simulink model "simulate_OFDM_basebandModulator"  (R2017a)
settings: Solver=VariableStepAuto  StartTime=0.0  StopTime=1  RelTol=1e-3
InitFcn:
  | Ts = 1/1000; % symbol time in serial data stream
  | N = 4; % number of orthogonal carriers
  | T = N*Ts; % symbol time in parallel data stream
libraries: commfilt2 x4, dspsrcs4 x4, commdigbbndpm3 x1, commrandsrc3 x1, dspindex x1
settings Model: Creator=prust  LastModifiedBy=prust

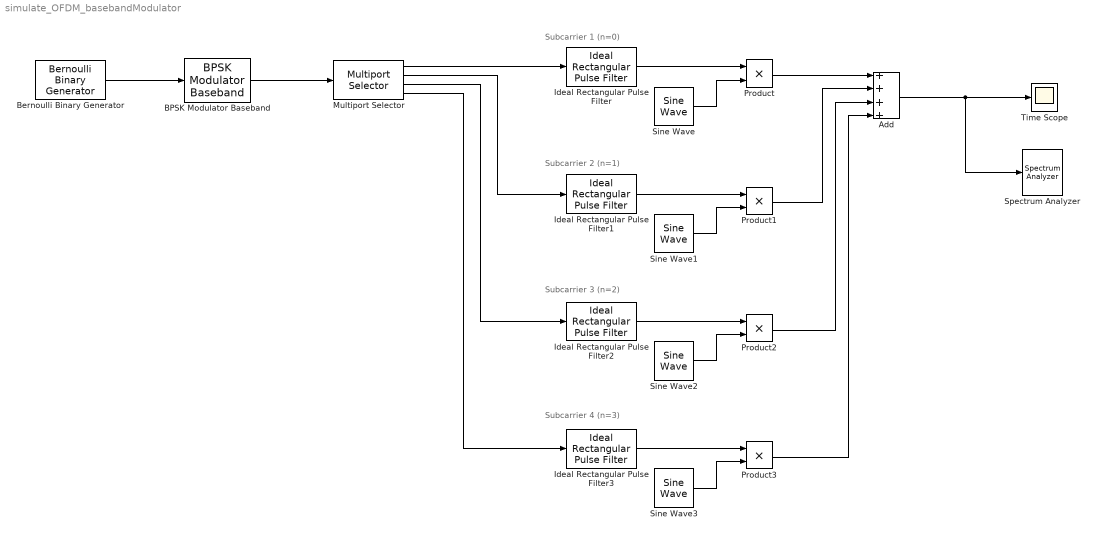
== system simulate_OFDM_basebandModulator ==
  note: Subcarrier 4 (n=3)
  note: Subcarrier 3 (n=2)
  note: Subcarrier 2 (n=1)
  note: Subcarrier 1 (n=0)
  Add : Sum  Inputs=4
  BPSK Modulator Baseband : commdigbbndpm3/BPSK Modulator Baseband  Ph=0  outDtype=double  outWordLen=16  outUDDataType=sfix(16)  outFracLenMode=Best precision  outFracLen=15  outDataTypeStr=double  outLastDataTypeStr=double
  Bernoulli Binary Generator : commrandsrc3/Bernoulli Binary Generator  ProbabilityOfZero=0.5  SeedSource=Auto  Seed=0  SampleTime=Ts  SamplesPerFrame=4  OutputDataType=double  SimulateUsing=Interpreted execution
  Ideal Rectangular Pulse Filter{,1..3} (4 alike) : commfilt2/Ideal Rectangular Pulse Filter  pulseLen=8  pulseDelay=0  InputProcessing=Columns as channels (frame based)  RateOptions=Enforce single-rate processing  sampMode=Mute  normCheck=off  normMode=Sum of samples  filterGain=1  saveAsFlag=0  roundingMode=Floor  overflowMode=off  firstCoeffDataTypeStr=Inherit: Same word length as input  firstCoeffMin=[]  firstCoeffMax=[]  firstCoeffLastDataTypeStr=Inherit: Same word length as input  outputDataTypeStr=Inherit: Same as accumulator  outputMin=[]  outputMax=[]  outputLastDataTypeStr=Inherit: Same as accumulator
      settings: SourceProductName=Communications System Toolbox  SourceProductBaseCode=CM
  Multiport Selector : dspindex/Multiport Selector  rowsOrCols=Rows  idxCellArray={ 1, 2, 3, 4 }  idxErrMode=Clip Index
  Product : Product
  "Product1 " : Product
  Product2 : Product
  Product3 : Product
  Sine Wave : dspsrcs4/Sine Wave  Amplitude=1  Frequency=-375  Phase=0  SampleMode=Discrete  OutComplex=Complex  CompMethod=Trigonometric fcn  TableSize=Speed  SampleTime=T/8  SamplesPerFrame=8  ResetState=Restart at time zero  OutputFrames=off  dataType=double  wordLen=16  udDataType=sfix(16)  fracBitsMode=Best precision  numFracBits=15  OutDataTypeStr=double  LastOutDataTypeStr=double
  Sine Wave1 : dspsrcs4/Sine Wave  Amplitude=1  Frequency=-125  Phase=0  SampleMode=Discrete  OutComplex=Complex  CompMethod=Trigonometric fcn  TableSize=Speed  SampleTime=T/8  SamplesPerFrame=8  ResetState=Restart at time zero  OutputFrames=off  dataType=double  wordLen=16  udDataType=sfix(16)  fracBitsMode=Best precision  numFracBits=15  OutDataTypeStr=double  LastOutDataTypeStr=double
  Sine Wave2 : dspsrcs4/Sine Wave  Amplitude=1  Frequency=125  Phase=0  SampleMode=Discrete  OutComplex=Complex  CompMethod=Trigonometric fcn  TableSize=Speed  SampleTime=T/8  SamplesPerFrame=8  ResetState=Restart at time zero  OutputFrames=off  dataType=double  wordLen=16  udDataType=sfix(16)  fracBitsMode=Best precision  numFracBits=15  OutDataTypeStr=double  LastOutDataTypeStr=double
  Sine Wave3 : dspsrcs4/Sine Wave  Amplitude=1  Frequency=375  Phase=0  SampleMode=Discrete  OutComplex=Complex  CompMethod=Trigonometric fcn  TableSize=Speed  SampleTime=T/8  SamplesPerFrame=8  ResetState=Restart at time zero  OutputFrames=off  dataType=double  wordLen=16  udDataType=sfix(16)  fracBitsMode=Best precision  numFracBits=15  OutDataTypeStr=double  LastOutDataTypeStr=double
  Spectrum Analyzer : SpectrumAnalyzer
  Time Scope : Scope
  wires:
  Bernoulli Binary Generator/1 -> BPSK Modulator Baseband/1
  Sine Wave1/1 -> "Product1 "/2
  Multiport Selector/2 -> Ideal Rectangular Pulse Filter1/1
  Multiport Selector/1 -> Ideal Rectangular Pulse Filter/1
  Sine Wave/1 -> Product/2
  Multiport Selector/3 -> Ideal Rectangular Pulse Filter2/1
  Sine Wave2/1 -> Product2/2
  Sine Wave3/1 -> Product3/2
  Multiport Selector/4 -> Ideal Rectangular Pulse Filter3/1
  Product/1 -> Add/1
  "Product1 "/1 -> Add/2
  Product2/1 -> Add/3
  Product3/1 -> Add/4
  Add/1 -> Time Scope/1, Spectrum Analyzer/1
  Ideal Rectangular Pulse Filter/1 -> Product/1
  Ideal Rectangular Pulse Filter1/1 -> "Product1 "/1
  Ideal Rectangular Pulse Filter2/1 -> Product2/1
  Ideal Rectangular Pulse Filter3/1 -> Product3/1
  BPSK Modulator Baseband/1 -> Multiport Selector/1
